simulink library "SingleWorkstationModelLibrary"  (R2014a)
settings: Solver=ode45  StartTime=0.0  StopTime=10.0  RelTol=1e-3
undefined symbols (not defined in the file or in its folder): se_randomizeseeds
(part 2 of 3)

== system SingleWorkstationModelLibrary/GGkWorkstation_MakeAndMoveBatches_Parallel ==
  note: % LICENSE: 3-clause "Revised" or "New" or "Modified" BSD License.
      | % Copyright (c) 2015, Georgia Institute of Technology.
      | % All rights reserved.
      | %
      | % Redistribution and use in source and binary forms, with or without
      | % modification, are permitted provided that the following conditions are met:
      | % * Redistributions of source code must retain the above copyright
      | % notice, this list of conditions and the following disclaimer.
      | % * Redistributions in binary form must reproduce the above copyright
      | % notice, this list of conditions and the following disclaimer in the
      | % documentation and/or other materials provided with the distribution.
      | % * Neither the name of the Georgia Institute of Technology nor the
      | % names of its contributors may be used to endorse or promote products
      | % derived from this software without specific prior written permission.
      | %
      | % THIS SOFTWARE IS PROVIDED BY THE COPYRIGHT HOLDERS AND CONTRIBUTORS "AS IS" AND
      | % ANY EXPRESS OR IMPLIED WARRANTIES, INCLUDING, BUT NOT LIMITED TO, THE IMPLIED
      | % WARRANTIES OF MERCHANTABILITY AND FITNESS FOR A PARTICULAR PURPOSE ARE
      | % DISCLAIMED. IN NO EVENT SHALL THE GEORGIA INSTITUTE OF TECHNOLOGY BE LIABLE FOR
      | % ANY DIRECT, INDIRECT, INCIDENTAL, SPECIAL, EXEMPLARY, OR CONSEQUENTIAL DAMAGES
      | % (INCLUDING, BUT NOT LIMITED TO, PROCUREMENT OF SUBSTITUTE GOODS OR SERVICES;
      | % LOSS OF USE, DATA, OR PROFITS; OR BUSINESS INTERRUPTION) HOWEVER CAUSED AND
      | % ON ANY THEORY OF LIABILITY, WHETHER IN CONTRACT, STRICT LIABILITY, OR TORT
      | % (INCLUDING NEGLIGENCE OR OTHERWISE) ARISING IN ANY WAY OUT OF THE USE OF THIS
      | % SOFTWARE, EVEN IF ADVISED OF THE POSSIBILITY OF SUCH DAMAGE.
  Clock : Clock
  ComputeTH : Subsystem
  ComputeWIP : Subsystem
  GGkWorkstation_MakeAndMoveBatches_Parallel : Subsystem  mask{MakeBatchSize=12, MoveBatchSize=1, NumberOfServers=1}
      mask prompts: MakeBatchSize "Make (a.k.a. Process) Batch Size:"; MoveBatchSize "Move (a.k.a. Transfer) Batch Size"; NumberOfServers "Number of servers:"
      mask Callback MakeBatchSize:
      | %% Capture pre-existing base workspace variables, to cleanup when done
      | preExistingVars = who;
      | 
      | 
      | %% MakeBatchSize is defined as a mask parameter
      | batchSizeStr = get_param(gcbh, 'MakeBatchSize');
      | batchSizeInt = int32(str2double(batchSizeStr));  %Enforce integer
      | if batchSizeInt < 1  %str2double returns NaN for non-numerical input, and int32 returns 0 for NaN
      |     error('Invalid input for MakeBatchSize');
      | end
      | set_param(gcbh, 'MakeBatchSize', num2str(batchSizeInt));  %Correct any non-integer value
      | 
      | 
      | %% Get paths of OutputSwitch, EntityCombiner, EntitySplitter, and PathCombiner
      | singleWksPath = [gcs '/' get(gcbh,'Name')];
      | outputSwitchPath = [singleWksPath '/MakeBatchOutputSwitch'];
      | entityCombinerPath = [singleWksPath '/MakeBatchEntityCombiner'];
      | entitySplitterPath = [singleWksPath '/MakeBatchEntitySplitter'];
      | pathCombinerPath = [singleWksPath '/MakeBatchPathCombiner'];
      | 
      | 
      | %% Unsure if needed:  Disable model library link to enable editing
      | %set_param(singleWksPath, 'LinkStatus', 'inactive');
      | 
      | 
      | %% Delete existing queues and connections
      | phOutputSwitch = get_param(outputSwitchPath, 'PortHandles');
      | phOutputSwitch = phOutputSwitch.RConn;
      | phEntityCombiner = get_param(entityCombinerPath, 'PortHandles');
      | phEntityCombiner = phEntityCombiner.LConn;
      | phEntitySplitter = get_param(entitySplitterPath, 'PortHandles');
      | phEntitySplitter = phEntitySplitter.RConn;
      | 
      | %Delete existing queues
      | oldBatchSize = get_param(outputSwitchPath, 'NumberOutputPorts');
      | queueNamesBeginWith = 'MakeBatchQ';  %Hard-codes a particular naming scheme
      | singleWksBlockList = get(gcbh, 'Blocks');
      | ECQueueMatches = strncmpi(queueNamesBeginWith, singleWksBlockList, length(queueNamesBeginWith));
      | ECQueueNames = singleWksBlockList(ECQueueMatches);
      | if ~isempty(ECQueueNames)
      |     for mm = 1 : length(ECQueueNames)
      |         queuePath = [singleWksPath '/' ECQueueNames{mm}];
      |         queueHandle = get_param(queuePath, 'Handle');
      |         delete(queueHandle);
      |     end
      | end
      | 
      | %Delete the lines
      | for iiiii = 1 : str2double(oldBatchSize)
      |     phOutputSwitchPos = get_param(phOutputSwitch(iiiii), 'Position');
      |     try delete_line(singleWksPath, phOutputSwitchPos); catch, end  %Fail silently
      |     phEntityCombinerPos = get_param(phEntityCombiner(iiiii), 'Position');
      |     try delete_line(singleWksPath, phEntityCombinerPos); catch, end  %Fail silently
      |     phEntitySplitterPos = get_param(phEntitySplitter(iiiii), 'Position');
      |     try delete_line(singleWksPath, phEntitySplitterPos); catch, end  %Fail silently
      | end
      | 
      | 
      | %% Set new number of ports
      | set_param(outputSwitchPath, 'NumberOutputPorts', batchSizeStr);
      | set_param(entityCombinerPath, 'NumberInputPorts', batchSizeStr);
      | set_param(entitySplitterPath, 'NumberOutputPorts', batchSizeStr);
      | set_param(pathCombinerPath, 'NumberInputPorts', batchSizeStr);
      | 
      | 
      | %% Add EntityCombiner input queues, plus connections between OutputSwitch and EntityCombiner
      | phOutputSwitch = get_param(outputSwitchPath, 'PortHandles');
      | phOutputSwitch = phOutputSwitch.RConn;
      | phEntityCombiner = get_param(entityCombinerPath, 'PortHandles');
      | phEntityCombiner = phEntityCombiner.LConn;
      | phEntitySplitter = get_param(entitySplitterPath, 'PortHandles');
      | phEntitySplitter = phEntitySplitter.RConn;
      | phPathCombiner = get_param(pathCombinerPath, 'PortHandles');
      | phPathCombiner = phPathCombiner.LConn;
      | 
      | queueLength = 80;
      | queueHeight = 20;
      | xOffset = 130;
      | prevBlockPos = get_param(outputSwitchPath, 'Position');
      | prevBlockHeight = prevBlockPos(4)-prevBlockPos(2);
      | yIncrement = prevBlockHeight / batchSizeInt;
      | for jjjjj = 1 : batchSizeInt
      |     queuePath = [singleWksPath '/' queueNamesBeginWith num2str(jjjjj)];
      |     queueHandle = add_block('built-in/FIFOQueue', queuePath);
      |     set_param(queueHandle, 'Capacity', 'Inf');  %Shouldn't be needed, but a good default
      | 
      |     left = prevBlockPos(1)+xOffset;
      |     top = double( prevBlockPos(2)+(jjjjj-1)*yIncrement );
      |     right = prevBlockPos(1)+xOffset+queueLength;
      |     bottom = double( prevBlockPos(2)+(jjjjj-1)*yIncrement+queueHeight );
      |     p = [left top right bottom];
      |     set_param(queueHandle, 'Position', p);  %Need a vector of doubles (not int32)
      | 
      |     QueuePortHandles = get_param(queueHandle, 'PortHandles');
      |     %Line from OutputSwitch to Queue
      |     OutputSwitchOutPortPos = get_param(phOutputSwitch(jjjjj), 'Position');
      |     QueueInPortPos = get_param(QueuePortHandles.LConn, 'Position');
      |     add_line(singleWksPath, [OutputSwitchOutPortPos; QueueInPortPos]);
      |     %Line from Queue to EntityCombiner
      |     QueueOutPortPos = get_param(QueuePortHandles.RConn, 'Position');
      |     EntityCombinerInPortPos = get_param(phEntityCombiner(jjjjj), 'Position');
      |     add_line(singleWksPath, [QueueOutPortPos; EntityCombinerInPortPos]);
      | end
      | 
      | 
      | %% Add connections between EntitySplitter and PathCombiner
      | for kkkkk = 1 : batchSizeInt
      |     phEntitySplitterPos = get_param(phEntitySplitter(kkkkk), 'Position');
      |     phPathCombinerPos = get_param(phPathCombiner(kkkkk), 'Position');
      |     add_line(singleWksPath, [phEntitySplitterPos; phPathCombinerPos]);
      | end
      | 
      | 
      | %% Cleanup, because mask callback executes in base workspace
      | clearvars('-except', preExistingVars{:});
      mask Callback MoveBatchSize:
      | %% Capture pre-existing base workspace variables, to cleanup when done
      | preExistingVars = who;
      | 
      | 
      | %% MoveBatchSize is defined as a mask parameter
      | batchSizeStr = get_param(gcbh, 'MoveBatchSize');
      | batchSizeInt = int32(str2double(batchSizeStr));  %Enforce integer
      | if batchSizeInt < 1  %str2double returns NaN for non-numerical input, and int32 returns 0 for NaN
      |     error('Invalid input for MoveBatchSize');
      | end
      | set_param(gcbh, 'MoveBatchSize', num2str(batchSizeInt));  %Correct any non-integer value
      | 
      | 
      | %% Get paths of OutputSwitch, EntityCombiner, EntitySplitter, and PathCombiner
      | singleWksPath = [gcs '/' get(gcbh,'Name')];
      | outputSwitchPath = [singleWksPath '/MoveBatchOutputSwitch'];
      | entityCombinerPath = [singleWksPath '/MoveBatchEntityCombiner'];
      | entitySplitterPath = [singleWksPath '/MoveBatchEntitySplitter'];
      | pathCombinerPath = [singleWksPath '/MoveBatchPathCombiner'];
      | 
      | 
      | %% Unsure if needed:  Disable model library link to enable editing
      | %set_param(singleWksPath, 'LinkStatus', 'inactive');
      | 
      | 
      | %% Delete existing queues and connections
      | phOutputSwitch = get_param(outputSwitchPath, 'PortHandles');
      | phOutputSwitch = phOutputSwitch.RConn;
      | phEntityCombiner = get_param(entityCombinerPath, 'PortHandles');
      | phEntityCombiner = phEntityCombiner.LConn;
      | phEntitySplitter = get_param(entitySplitterPath, 'PortHandles');
      | phEntitySplitter = phEntitySplitter.RConn;
      | 
      | %Delete existing queues
      | oldBatchSize = get_param(outputSwitchPath, 'NumberOutputPorts');
      | queueNamesBeginWith = 'MoveBatchQ';  %Hard-codes a particular naming scheme
      | singleWksBlockList = get(gcbh, 'Blocks');
      | ECQueueMatches = strncmpi(queueNamesBeginWith, singleWksBlockList, length(queueNamesBeginWith));
      | ECQueueNames = singleWksBlockList(ECQueueMatches);
      | if ~isempty(ECQueueNames)
      |     for mm = 1 : length(ECQueueNames)
      |         queuePath = [singleWksPath '/' ECQueueNames{mm}];
      |         queueHandle = get_param(queuePath, 'Handle');
      |         delete(queueHandle);
      |     end
      | end
      | 
      | %Delete the lines
      | for iiiii = 1 : str2double(oldBatchSize)
      |     phOutputSwitchPos = get_param(phOutputSwitch(iiiii), 'Position');
      |     try delete_line(singleWksPath, phOutputSwitchPos); catch, end  %Fail silently
      |     phEntityCombinerPos = get_param(phEntityCombiner(iiiii), 'Position');
      |     try delete_line(singleWksPath, phEntityCombinerPos); catch, end  %Fail silently
      |     phEntitySplitterPos = get_param(phEntitySplitter(iiiii), 'Position');
      |     try delete_line(singleWksPath, phEntitySplitterPos); catch, end  %Fail silently
      | end
      | 
      | 
      | %% Set new number of ports
      | set_param(outputSwitchPath, 'NumberOutputPorts', batchSizeStr);
      | set_param(entityCombinerPath, 'NumberInputPorts', batchSizeStr);
      | set_param(entitySplitterPath, 'NumberOutputPorts', batchSizeStr);
      | set_param(pathCombinerPath, 'NumberInputPorts', batchSizeStr);
      | 
      | 
      | %% Add EntityCombiner input queues, plus connections between OutputSwitch and EntityCombiner
      | phOutputSwitch = get_param(outputSwitchPath, 'PortHandles');
      | phOutputSwitch = phOutputSwitch.RConn;
      | phEntityCombiner = get_param(entityCombinerPath, 'PortHandles');
      | phEntityCombiner = phEntityCombiner.LConn;
      | phEntitySplitter = get_param(entitySplitterPath, 'PortHandles');
      | phEntitySplitter = phEntitySplitter.RConn;
      | phPathCombiner = get_param(pathCombinerPath, 'PortHandles');
      | phPathCombiner = phPathCombiner.LConn;
      | 
      | queueLength = 80;
      | queueHeight = 20;
      | xOffset = 130;
      | prevBlockPos = get_param(outputSwitchPath, 'Position');
      | prevBlockHeight = prevBlockPos(4)-prevBlockPos(2);
      | yIncrement = prevBlockHeight / batchSizeInt;
      | for jjjjj = 1 : batchSizeInt
      |     queuePath = [singleWksPath '/' queueNamesBeginWith num2str(jjjjj)];
      |     queueHandle = add_block('built-in/FIFOQueue', queuePath);
      |     set_param(queueHandle, 'Capacity', 'Inf');
      | 
      | 	left = prevBlockPos(1)+xOffset;
      |     top = double( prevBlockPos(2)+(jjjjj-1)*yIncrement );
      |     right = prevBlockPos(1)+xOffset+queueLength;
      |     bottom = double( prevBlockPos(2)+(jjjjj-1)*yIncrement+queueHeight );
      |     p = [left top right bottom];
      |     set_param(queueHandle, 'Position', p);  %Need a vector of doubles (not int32)
      | 
      |     QueuePortHandles = get_param(queueHandle, 'PortHandles');
      |     %Line from OutputSwitch to Queue
      |     OutputSwitchOutPortPos = get_param(phOutputSwitch(jjjjj), 'Position');
      |     QueueInPortPos = get_param(QueuePortHandles.LConn, 'Position');
      |     add_line(singleWksPath, [OutputSwitchOutPortPos; QueueInPortPos]);
      |     %Line from Queue to EntityCombiner
      |     QueueOutPortPos = get_param(QueuePortHandles.RConn, 'Position');
      |     EntityCombinerInPortPos = get_param(phEntityCombiner(jjjjj), 'Position');
      |     add_line(singleWksPath, [QueueOutPortPos; EntityCombinerInPortPos]);
      | end
      | 
      | 
      | %% Add connections between EntitySplitter and PathCombiner
      | for kkkkk = 1 : batchSizeInt
      |     phEntitySplitterPos = get_param(phEntitySplitter(kkkkk), 'Position');
      |     phPathCombinerPos = get_param(phPathCombiner(kkkkk), 'Position');
      |     add_line(singleWksPath, [phEntitySplitterPos; phPathCombinerPos]);
      | end
      | 
      | 
      | %% Cleanup, because mask callback executes in base workspace
      | clearvars('-except', preExistingVars{:});
      mask TypeOptions NumberOfServers: N-Server/NumberOfServers
      mask DialogControl DescTextVar Prompt: GGk Workstation with Make and Move Batches.  This model implements parallel batch processing, meaning Processing Time is for an entire make (a.k.a. process) batch.  Tokens are output only after a full move (a.k.a. transfer) batch is assembled, and are output individually (as individual entities, not as a batch entity).
  RandomNumbers_ProcessingTimes : EventBasedRandomNumber  meanExp=90  minUnif=40  maxUnif=40  pOneBern=40  pSuccessBino=40  numTrialBino=40  minTri=40  maxTri=40  modeTri=40  thresholdGam=40  scaleGam=40  shapeGam=40  meanNorm=90  stdNorm=eps  pSuccessGeo=40  meanPoiss=40  thresholdLogn=40  scaleLogn=40  shapeLogn=40  thresholdLogl=40  scaleLogl=40  minBeta=40  maxBeta=40  shape1Beta=40  shape2Beta=40  minUnid=40  maxUnid=40  numValueUnid=40  thresholdWbl=40  scaleWbl=40  shapeWbl=40  valueVecCont=40  cdfVecCont=40  valueVecDisc=40  probVecDisc=40  Seed=42055
  Arrivals : PMIOPort  Port=1  Side=Left
  Departures : PMIOPort  Port=2  Side=Right
  WIP_samples : Outport
  WIP_average : Outport  Port=2
  CT_samples : Outport  Port=3
  CT_average : Outport  Port=4
  TH_samples : Outport  Port=5
  TH_average : Outport  Port=6
  Util_average : Outport  Port=7
  wires:
  GGkWorkstation_MakeAndMoveBatches_Parallel/5(Util_average) -> Util_average/1
  GGkWorkstation_MakeAndMoveBatches_Parallel/2(nDepartures) -> ComputeWIP/2(nDepartures), ComputeTH/2(nDepartures)
  GGkWorkstation_MakeAndMoveBatches_Parallel/3(CT_samples) -> CT_samples/1
  GGkWorkstation_MakeAndMoveBatches_Parallel/4(CT_average) -> CT_average/1
  ComputeWIP/1(WIP_samples) -> WIP_samples/1
  ComputeWIP/2(WIP_average) -> WIP_average/1
  GGkWorkstation_MakeAndMoveBatches_Parallel/1(nArrivals) -> ComputeWIP/1(nArrivals)
  Clock/1 -> ComputeWIP/3(CurrentTime), ComputeTH/1(CurrentTime)
  ComputeTH/1(TH_average) -> TH_average/1
  ComputeTH/2(TH_samples) -> TH_samples/1
  RandomNumbers_ProcessingTimes/1 -> GGkWorkstation_MakeAndMoveBatches_Parallel/1(ProcessingTimes)
  connections:
  Departures/RConn1 -- GGkWorkstation_MakeAndMoveBatches_Parallel/RConn1
  GGkWorkstation_MakeAndMoveBatches_Parallel/LConn1 -- Arrivals/RConn1

== system SingleWorkstationModelLibrary/GG1Workstation_FailuresAndSetups/ComputeTH ==
  CurrentTime : Inport
  nDepartures : Inport  Port=2
  Derivative : Derivative
  Divide1 : Product  Inputs=/*
  Event to Timed Signal1 : EventToTimedSignal
  TH_average : Outport
  TH_samples : Outport  Port=2
  wires:
  CurrentTime/1 -> Divide1/1
  Event to Timed Signal1/1 -> Derivative/1, Divide1/2
  Divide1/1 -> TH_average/1
  Derivative/1 -> TH_samples/1
  nDepartures/1 -> Event to Timed Signal1/1

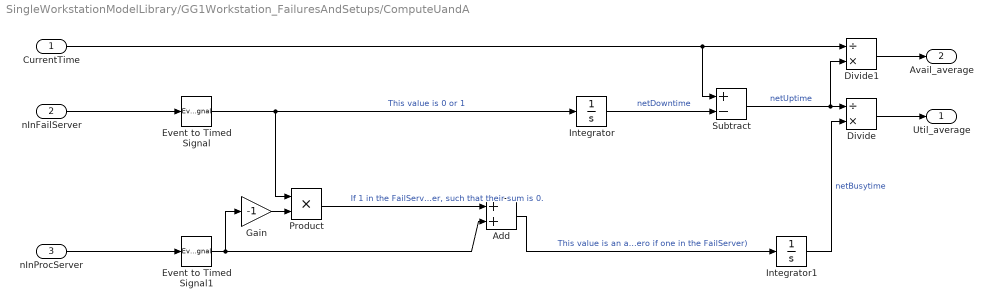
== system SingleWorkstationModelLibrary/GG1Workstation_FailuresAndSetups/ComputeUandA ==
  CurrentTime : Inport
  nInFailServer : Inport  Port=2
  nInProcServer : Inport  Port=3
  Add : Sum
  Divide : Product  Inputs=/*
  Divide1 : Product  Inputs=/*
  Event to Timed Signal : EventToTimedSignal
  Event to Timed Signal1 : EventToTimedSignal
  Gain : Gain  Gain=-1
  Integrator : Integrator
  Integrator1 : Integrator
  Product : Product
  Subtract : Sum  Inputs=+-
  Util_average : Outport
  Avail_average : Outport  Port=2
  wires:
  Event to Timed Signal/1 -> Integrator/1, Product/1  "This value is 0 or 1"
  nInFailServer/1 -> Event to Timed Signal/1
  nInProcServer/1 -> Event to Timed Signal1/1
  Integrator/1 -> Subtract/2  "netDowntime"
  CurrentTime/1 -> Subtract/1, Divide1/1
  Divide/1 -> Util_average/1
  Subtract/1 -> Divide/1, Divide1/2  "netUptime"
  Integrator1/1 -> Divide/2  "netBusytime"
  Gain/1 -> Product/2
  Product/1 -> Add/1  "If 1 in the FailServer, then this value should be negative the number in the ProcServer, such that their sum is 0."
  Add/1 -> Integrator1/1  "This value is an adjusted number in the ProcServer (zero if one in the FailServer)"
  Event to Timed Signal1/1 -> Add/2, Gain/1
  Divide1/1 -> Avail_average/1

== system SingleWorkstationModelLibrary/GG1Workstation_FailuresAndSetups/ComputeWIP ==
  nArrivals : Inport
  nDepartures : Inport  Port=2
  CurrentTime : Inport  Port=3
  Divide : Product  Inputs=*/
  Event to Timed Signal : EventToTimedSignal
  Integrator : Integrator
  Subtract : Sum  Inputs=+-
  WIP_samples : Outport
  WIP_average : Outport  Port=2
  wires:
  Subtract/1 -> WIP_samples/1, Event to Timed Signal/1
  Event to Timed Signal/1 -> Integrator/1
  Divide/1 -> WIP_average/1
  Integrator/1 -> Divide/1
  nArrivals/1 -> Subtract/1
  nDepartures/1 -> Subtract/2
  CurrentTime/1 -> Divide/2

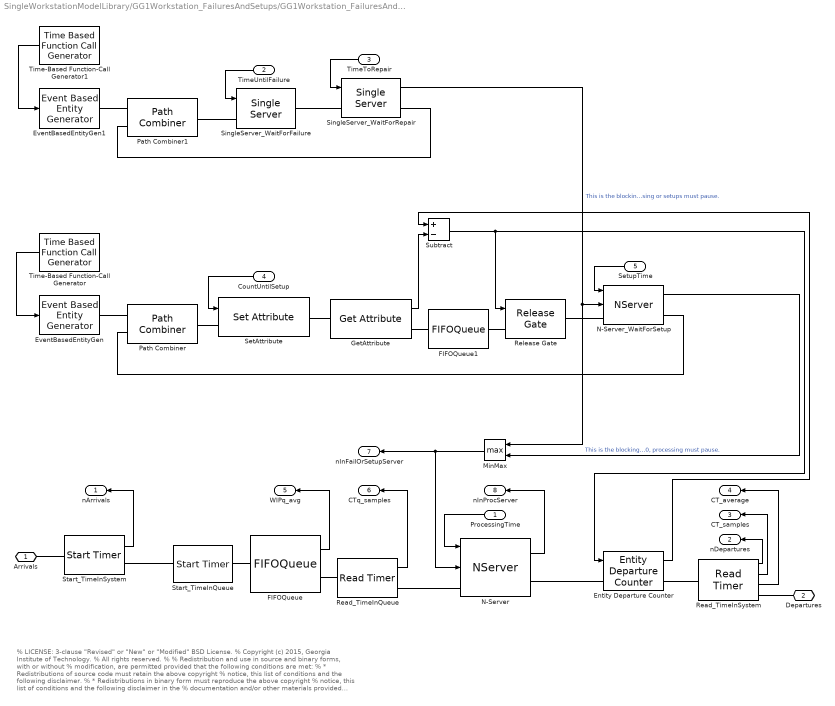
== system SingleWorkstationModelLibrary/GG1Workstation_FailuresAndSetups/GG1Workstation_FailuresAndSetups ==
  note: % LICENSE: 3-clause "Revised" or "New" or "Modified" BSD License.
      | % Copyright (c) 2015, Georgia Institute of Technology.
      | % All rights reserved.
      | %
      | % Redistribution and use in source and binary forms, with or without
      | % modification, are permitted provided that the following conditions are met:
      | % * Redistributions of source code must retain the above copyright
      | % notice, this list of conditions and the following disclaimer.
      | % * Redistributions in binary form must reproduce the above copyright
      | % notice, this list of conditions and the following disclaimer in the
      | % documentation and/or other materials provided with the distribution.
      | % * Neither the name of the Georgia Institute of Technology nor the
      | % names of its contributors may be used to endorse or promote products
      | % derived from this software without specific prior written permission.
      | %
      | % THIS SOFTWARE IS PROVIDED BY THE COPYRIGHT HOLDERS AND CONTRIBUTORS "AS IS" AND
      | % ANY EXPRESS OR IMPLIED WARRANTIES, INCLUDING, BUT NOT LIMITED TO, THE IMPLIED
      | % WARRANTIES OF MERCHANTABILITY AND FITNESS FOR A PARTICULAR PURPOSE ARE
      | % DISCLAIMED. IN NO EVENT SHALL THE GEORGIA INSTITUTE OF TECHNOLOGY BE LIABLE FOR
      | % ANY DIRECT, INDIRECT, INCIDENTAL, SPECIAL, EXEMPLARY, OR CONSEQUENTIAL DAMAGES
      | % (INCLUDING, BUT NOT LIMITED TO, PROCUREMENT OF SUBSTITUTE GOODS OR SERVICES;
      | % LOSS OF USE, DATA, OR PROFITS; OR BUSINESS INTERRUPTION) HOWEVER CAUSED AND
      | % ON ANY THEORY OF LIABILITY, WHETHER IN CONTRACT, STRICT LIABILITY, OR TORT
      | % (INCLUDING NEGLIGENCE OR OTHERWISE) ARISING IN ANY WAY OUT OF THE USE OF THIS
      | % SOFTWARE, EVEN IF ADVISED OF THE POSSIBILITY OF SUCH DAMAGE.
  ProcessingTime : Inport
  TimeUntilFailure : Inport  Port=2
  TimeToRepair : Inport  Port=3
  CountUntilSetup : Inport  Port=4
  SetupTime : Inport  Port=5
  Entity Departure Counter : EntityDepartureCounter  NumberDepartedToSignal=on  NumberDepartedToAttribute=off  CounterResetTypeOption=Trigger from port tr
  EventBasedEntityGen : EventBasedEntityGenerator  GenerateEntitiesUpon=Function call from port fcn
  EventBasedEntityGen1 : EventBasedEntityGenerator  GenerateEntitiesUpon=Function call from port fcn
  FIFOQueue : FIFOQueue  Capacity=Capacity  StatAverageQueueLength=on
      settings: OutputPortMap=o3
  FIFOQueue1 : FIFOQueue  Capacity=Inf
  GetAttribute : GetAttribute  AttributeName=CountUntilSetup  EvaluatedDefaultAttributeValue={ []}
      settings: OutputPortMap=o1
  MinMax : MinMax  Function=max  Inputs=2
  N-Server : NServer  NumberOfServers=1  ServiceTimeFrom=Signal port t  AllowServiceControl=on  BlockWhileSignalOn=on  StatNumberInBlock=on
      settings: InputPortMap=u0,u1  OutputPortMap=o1
  N-Server_WaitForSetup : NServer  NumberOfServers=1  ServiceTimeFrom=Signal port t  AllowServiceControl=on  BlockWhileSignalOn=on  StatNumberInBlock=on
      settings: InputPortMap=u0,u1  OutputPortMap=o1
  Path Combiner : PathCombiner  NumberInputPorts=2
  Path Combiner1 : PathCombiner  NumberInputPorts=2
  Read_TimeInQueue : ReadTimer  TimerTag=TimeInQueue  StatTimeElapsed=on
      settings: OutputPortMap=o2
  Read_TimeInSystem : ReadTimer  TimerTag=TimeInSystem  StatNumberDeparted=on  StatTimeElapsed=on  StatAverageTimeElapsed=on
      settings: OutputPortMap=o0,o2,o3
  Release Gate : ReleaseGate  OpenGateUpon=Trigger from port tr
  SetAttribute : SetAttribute  AttributeName=CountUntilSetup  AttributeFrom=Signal port  EvaluatedAttributeValue={ []}
  SingleServer_WaitForFailure : SingleServer  ServiceTimeFrom=Signal port t  AttributeName=TimeUntilFailure
  SingleServer_WaitForRepair : SingleServer  ServiceTimeFrom=Signal port t  AttributeName=TimeToRepair  StatNumberInBlock=on
      settings: OutputPortMap=o1
  Start_TimeInQueue : StartTimer  TimerTag=TimeInQueue  TimerStartedOption=Restart
  Start_TimeInSystem : StartTimer  TimerTag=TimeInSystem  TimerStartedOption=Restart  StatNumberDeparted=on
  Subtract : Sum  Inputs=+-
  Time-Based Function-Call Generator : TimeBasedFunctionCallGenerator  EventGenerationMode=Only at simulation start
  Time-Based Function-Call Generator1 : TimeBasedFunctionCallGenerator  EventGenerationMode=Only at simulation start
  Arrivals : PMIOPort  Port=1  Side=Left
  Departures : PMIOPort  Port=2  Side=Right
  nArrivals : Outport
  nDepartures : Outport  Port=2
  CT_samples : Outport  Port=3
  CT_average : Outport  Port=4
  WIPq_avg : Outport  Port=5
  CTq_samples : Outport  Port=6
  nInFailOrSetupServer : Outport  Port=7
  nInProcServer : Outport  Port=8
  wires:
  Read_TimeInSystem/2 -> CT_samples/1
  Read_TimeInQueue/1 -> CTq_samples/1
  FIFOQueue/1 -> WIPq_avg/1
  Start_TimeInSystem/1 -> nArrivals/1
  Read_TimeInSystem/1 -> nDepartures/1
  ProcessingTime/1 -> N-Server/1
  Read_TimeInSystem/3 -> CT_average/1
  Time-Based Function-Call Generator/1 -> EventBasedEntityGen/1
  CountUntilSetup/1 -> SetAttribute/1
  Subtract/1 -> Release Gate/1, Entity Departure Counter/1
  GetAttribute/1 -> Subtract/2
  Entity Departure Counter/1 -> Subtract/1
  N-Server/1 -> nInProcServer/1
  SetupTime/1 -> N-Server_WaitForSetup/1
  Time-Based Function-Call Generator1/1 -> EventBasedEntityGen1/1
  TimeToRepair/1 -> SingleServer_WaitForRepair/1
  TimeUntilFailure/1 -> SingleServer_WaitForFailure/1
  SingleServer_WaitForRepair/1 -> MinMax/1, N-Server_WaitForSetup/2  "This is the blocking signal from failures. When >0, processing or setups must pause."
  N-Server_WaitForSetup/1 -> MinMax/2  "This is the blocking signal from setups.  When >0, processing must pause."
  MinMax/1 -> nInFailOrSetupServer/1, N-Server/2
  connections:
  Arrivals/RConn1 -- Start_TimeInSystem/LConn1
  FIFOQueue/RConn1 -- Read_TimeInQueue/LConn1
  Start_TimeInSystem/RConn1 -- Start_TimeInQueue/LConn1
  Read_TimeInSystem/RConn1 -- Departures/RConn1
  Read_TimeInQueue/RConn1 -- N-Server/LConn1
  Start_TimeInQueue/RConn1 -- FIFOQueue/LConn1
  Path Combiner/RConn1 -- SetAttribute/LConn1
  EventBasedEntityGen/RConn1 -- Path Combiner/LConn1
  Path Combiner/LConn2 -- N-Server_WaitForSetup/RConn1
  N-Server/RConn1 -- Entity Departure Counter/LConn1
  Entity Departure Counter/RConn1 -- Read_TimeInSystem/LConn1
  FIFOQueue1/LConn1 -- GetAttribute/RConn1
  N-Server_WaitForSetup/LConn1 -- Release Gate/RConn1
  FIFOQueue1/RConn1 -- Release Gate/LConn1
  SetAttribute/RConn1 -- GetAttribute/LConn1
  Path Combiner1/LConn2 -- SingleServer_WaitForRepair/RConn1
  SingleServer_WaitForRepair/LConn1 -- SingleServer_WaitForFailure/RConn1
  EventBasedEntityGen1/RConn1 -- Path Combiner1/LConn1
  Path Combiner1/RConn1 -- SingleServer_WaitForFailure/LConn1

== system SingleWorkstationModelLibrary/GG1Workstation_MakeAndMoveBatches_SerialWithSetups/ComputeTH ==
  CurrentTime : Inport
  nDepartures : Inport  Port=2
  Derivative : Derivative
  Divide1 : Product  Inputs=/*
  Event to Timed Signal1 : EventToTimedSignal
  TH_average : Outport
  TH_samples : Outport  Port=2
  wires:
  CurrentTime/1 -> Divide1/1
  Event to Timed Signal1/1 -> Derivative/1, Divide1/2
  Divide1/1 -> TH_average/1
  Derivative/1 -> TH_samples/1
  nDepartures/1 -> Event to Timed Signal1/1

== system SingleWorkstationModelLibrary/GG1Workstation_MakeAndMoveBatches_SerialWithSetups/ComputeWIP ==
  nArrivals : Inport
  nDepartures : Inport  Port=2
  CurrentTime : Inport  Port=3
  Divide : Product  Inputs=*/
  Event to Timed Signal : EventToTimedSignal
  Integrator : Integrator
  Subtract : Sum  Inputs=+-
  WIP_samples : Outport
  WIP_average : Outport  Port=2
  wires:
  Subtract/1 -> WIP_samples/1, Event to Timed Signal/1
  Event to Timed Signal/1 -> Integrator/1
  Divide/1 -> WIP_average/1
  Integrator/1 -> Divide/1
  nArrivals/1 -> Subtract/1
  nDepartures/1 -> Subtract/2
  CurrentTime/1 -> Divide/2

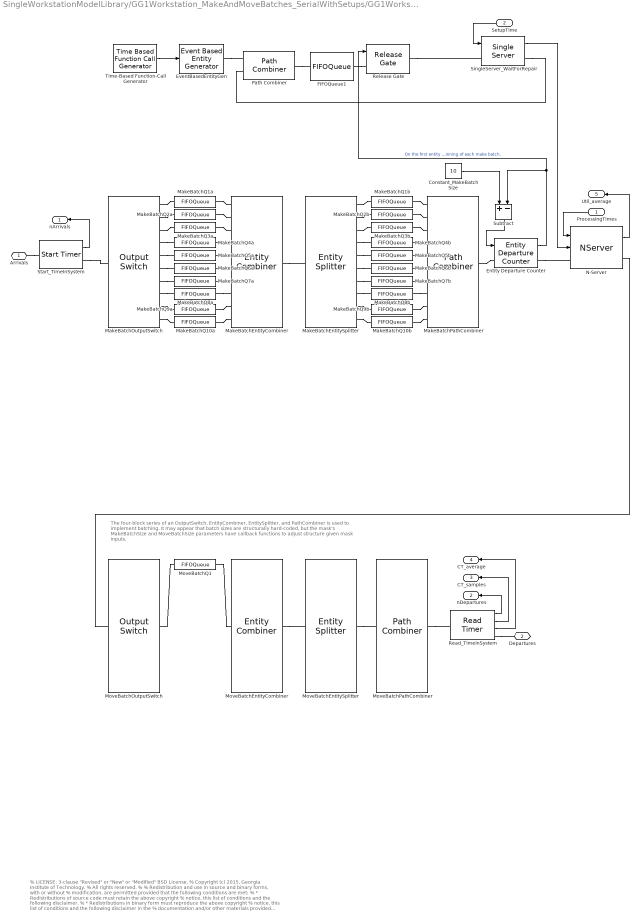
== system SingleWorkstationModelLibrary/GG1Workstation_MakeAndMoveBatches_SerialWithSetups/GG1Workstation_MakeAndMoveBatches_SerialWithSetups ==
  note: The four-block series of an OutputSwitch, EntityCombiner, EntitySplitter, and PathCombiner is used
      | to implement batching. It may appear that batch sizes are structurally hard-coded, but the mask's
      | MakeBatchSize and MoveBatchSize parameters have callback functions to adjust structure given
      | mask inputs.
  note: % LICENSE: 3-clause "Revised" or "New" or "Modified" BSD License.
      | % Copyright (c) 2015, Georgia Institute of Technology.
      | % All rights reserved.
      | %
      | % Redistribution and use in source and binary forms, with or without
      | % modification, are permitted provided that the following conditions are met:
      | % * Redistributions of source code must retain the above copyright
      | % notice, this list of conditions and the following disclaimer.
      | % * Redistributions in binary form must reproduce the above copyright
      | % notice, this list of conditions and the following disclaimer in the
      | % documentation and/or other materials provided with the distribution.
      | % * Neither the name of the Georgia Institute of Technology nor the
      | % names of its contributors may be used to endorse or promote products
      | % derived from this software without specific prior written permission.
      | %
      | % THIS SOFTWARE IS PROVIDED BY THE COPYRIGHT HOLDERS AND CONTRIBUTORS "AS IS" AND
      | % ANY EXPRESS OR IMPLIED WARRANTIES, INCLUDING, BUT NOT LIMITED TO, THE IMPLIED
      | % WARRANTIES OF MERCHANTABILITY AND FITNESS FOR A PARTICULAR PURPOSE ARE
      | % DISCLAIMED. IN NO EVENT SHALL THE GEORGIA INSTITUTE OF TECHNOLOGY BE LIABLE FOR
      | % ANY DIRECT, INDIRECT, INCIDENTAL, SPECIAL, EXEMPLARY, OR CONSEQUENTIAL DAMAGES
      | % (INCLUDING, BUT NOT LIMITED TO, PROCUREMENT OF SUBSTITUTE GOODS OR SERVICES;
      | % LOSS OF USE, DATA, OR PROFITS; OR BUSINESS INTERRUPTION) HOWEVER CAUSED AND
      | % ON ANY THEORY OF LIABILITY, WHETHER IN CONTRACT, STRICT LIABILITY, OR TORT
      | % (INCLUDING NEGLIGENCE OR OTHERWISE) ARISING IN ANY WAY OUT OF THE USE OF THIS
      | % SOFTWARE, EVEN IF ADVISED OF THE POSSIBILITY OF SUCH DAMAGE.
  ProcessingTimes : Inport
  SetupTime : Inport  Port=2
  Constant_MakeBatchSize : Constant  Value=10
  Entity Departure Counter : EntityDepartureCounter  NumberDepartedToSignal=on  NumberDepartedToAttribute=off  CounterResetTypeOption=Trigger from port tr  CounterResetEdgeOption=Falling
  EventBasedEntityGen : EventBasedEntityGenerator  GenerateEntitiesUpon=Function call from port fcn
  FIFOQueue1 : FIFOQueue  Capacity=Inf
  MakeBatchEntityCombiner : EntityCombiner  NumberInputPorts=10  AttributeAccessibility=off  TimerAccessibility=off
  MakeBatchEntitySplitter : EntitySplitter  NumberOutputPorts=10
  MakeBatchOutputSwitch : OutputSwitch  NumberOutputPorts=10  SwitchingCriterion=Round robin
  MakeBatchPathCombiner : PathCombiner  NumberInputPorts=10
  MakeBatchQ10a : FIFOQueue  Capacity=Inf
  MakeBatchQ10b : FIFOQueue  Capacity=1
  MakeBatchQ1a : FIFOQueue  Capacity=Inf
  MakeBatchQ1b : FIFOQueue  Capacity=1
  MakeBatchQ2a : FIFOQueue  Capacity=Inf
  MakeBatchQ2b : FIFOQueue  Capacity=1
  MakeBatchQ3a : FIFOQueue  Capacity=Inf
  MakeBatchQ3b : FIFOQueue  Capacity=1
  MakeBatchQ4a : FIFOQueue  Capacity=Inf
  MakeBatchQ4b : FIFOQueue  Capacity=1
  MakeBatchQ5a : FIFOQueue  Capacity=Inf
  MakeBatchQ5b : FIFOQueue  Capacity=1
  MakeBatchQ6a : FIFOQueue  Capacity=Inf
  MakeBatchQ6b : FIFOQueue  Capacity=1
  MakeBatchQ7a : FIFOQueue  Capacity=Inf
  MakeBatchQ7b : FIFOQueue  Capacity=1
  MakeBatchQ8a : FIFOQueue  Capacity=Inf
  MakeBatchQ8b : FIFOQueue  Capacity=1
  MakeBatchQ9a : FIFOQueue  Capacity=Inf
  MakeBatchQ9b : FIFOQueue  Capacity=1
  MoveBatchEntityCombiner : EntityCombiner  NumberInputPorts=1  AttributeAccessibility=off  TimerAccessibility=off
  MoveBatchEntitySplitter : EntitySplitter  NumberOutputPorts=1
  MoveBatchOutputSwitch : OutputSwitch  NumberOutputPorts=1  SwitchingCriterion=Round robin
  MoveBatchPathCombiner : PathCombiner  NumberInputPorts=1
  MoveBatchQ1 : FIFOQueue  Capacity=1
  N-Server : NServer  NumberOfServers=1  ServiceTimeFrom=Signal port t  AllowServiceControl=on  StatUtilization=on
      settings: InputPortMap=u0,u1  OutputPortMap=o5
  Path Combiner : PathCombiner  NumberInputPorts=2
  Read_TimeInSystem : ReadTimer  TimerTag=TimeInSystem  StatNumberDeparted=on  StatTimeElapsed=on  StatAverageTimeElapsed=on
      settings: OutputPortMap=o0,o2,o3
  Release Gate : ReleaseGate  OpenGateUpon=Trigger from port tr
  SingleServer_WaitForRepair : SingleServer  ServiceTimeFrom=Signal port t  AttributeName=SetupTime  StatNumberInBlock=on
      settings: OutputPortMap=o1
  Start_TimeInSystem : StartTimer  TimerTag=TimeInSystem  TimerStartedOption=Restart  StatNumberDeparted=on
  Subtract : Sum  Inputs=+-
  Time-Based Function-Call Generator : TimeBasedFunctionCallGenerator  EventGenerationMode=Only at simulation start
  Arrivals : PMIOPort  Port=1  Side=Left
  Departures : PMIOPort  Port=2  Side=Right
  nArrivals : Outport
  nDepartures : Outport  Port=2
  CT_samples : Outport  Port=3
  CT_average : Outport  Port=4
  Util_average : Outport  Port=5
  wires:
  Start_TimeInSystem/1 -> nArrivals/1
  Read_TimeInSystem/1 -> nDepartures/1
  Read_TimeInSystem/2 -> CT_samples/1
  ProcessingTimes/1 -> N-Server/1
  Read_TimeInSystem/3 -> CT_average/1
  Time-Based Function-Call Generator/1 -> EventBasedEntityGen/1
  SingleServer_WaitForRepair/1 -> N-Server/2
  SetupTime/1 -> SingleServer_WaitForRepair/1
  Entity Departure Counter/1 -> Subtract/2, Release Gate/1  "On the first entity of a make batch, this signal rises from 0 to 1 and triggers the release of a setup entity. The effect is setups which are not count-based, but rather upon the beginning of each make batch."
  Constant_MakeBatchSize/1 -> Subtract/1
  Subtract/1 -> Entity Departure Counter/1
  N-Server/1 -> Util_average/1
  connections:
  Read_TimeInSystem/RConn1 -- Departures/RConn1
  Arrivals/RConn1 -- Start_TimeInSystem/LConn1
  MoveBatchEntityCombiner/RConn1 -- MoveBatchEntitySplitter/LConn1
  Start_TimeInSystem/RConn1 -- MakeBatchOutputSwitch/LConn1
  MoveBatchPathCombiner/RConn1 -- Read_TimeInSystem/LConn1
  EventBasedEntityGen/RConn1 -- Path Combiner/LConn1
  SingleServer_WaitForRepair/RConn1 -- Path Combiner/LConn2
  Release Gate/RConn1 -- SingleServer_WaitForRepair/LConn1
  FIFOQueue1/RConn1 -- Release Gate/LConn1
  MakeBatchEntityCombiner/RConn1 -- MakeBatchEntitySplitter/LConn1
  Path Combiner/RConn1 -- FIFOQueue1/LConn1
  MakeBatchPathCombiner/RConn1 -- Entity Departure Counter/LConn1
  Entity Departure Counter/RConn1 -- N-Server/LConn1
  N-Server/RConn1 -- MoveBatchOutputSwitch/LConn1
  MakeBatchOutputSwitch/RConn1 -- MakeBatchQ1a/LConn1
  MakeBatchQ1a/RConn1 -- MakeBatchEntityCombiner/LConn1
  MakeBatchEntitySplitter/RConn1 -- MakeBatchQ1b/LConn1
  MakeBatchQ1b/RConn1 -- MakeBatchPathCombiner/LConn1
  MakeBatchOutputSwitch/RConn2 -- MakeBatchQ2a/LConn1
  MakeBatchQ2a/RConn1 -- MakeBatchEntityCombiner/LConn2
  MakeBatchEntitySplitter/RConn2 -- MakeBatchQ2b/LConn1
  MakeBatchQ2b/RConn1 -- MakeBatchPathCombiner/LConn2
  MakeBatchOutputSwitch/RConn3 -- MakeBatchQ3a/LConn1
  MakeBatchQ3a/RConn1 -- MakeBatchEntityCombiner/LConn3
  MakeBatchEntitySplitter/RConn3 -- MakeBatchQ3b/LConn1
  MakeBatchQ3b/RConn1 -- MakeBatchPathCombiner/LConn3
  MakeBatchOutputSwitch/RConn4 -- MakeBatchQ4a/LConn1
  MakeBatchQ4a/RConn1 -- MakeBatchEntityCombiner/LConn4
  MakeBatchEntitySplitter/RConn4 -- MakeBatchQ4b/LConn1
  MakeBatchQ4b/RConn1 -- MakeBatchPathCombiner/LConn4
  MakeBatchOutputSwitch/RConn5 -- MakeBatchQ5a/LConn1
  MakeBatchQ5a/RConn1 -- MakeBatchEntityCombiner/LConn5
  MakeBatchEntitySplitter/RConn5 -- MakeBatchQ5b/LConn1
  MakeBatchQ5b/RConn1 -- MakeBatchPathCombiner/LConn5
  MakeBatchOutputSwitch/RConn6 -- MakeBatchQ6a/LConn1
  MakeBatchQ6a/RConn1 -- MakeBatchEntityCombiner/LConn6
  MakeBatchEntitySplitter/RConn6 -- MakeBatchQ6b/LConn1
  MakeBatchQ6b/RConn1 -- MakeBatchPathCombiner/LConn6
  MakeBatchOutputSwitch/RConn7 -- MakeBatchQ7a/LConn1
  MakeBatchQ7a/RConn1 -- MakeBatchEntityCombiner/LConn7
  MakeBatchEntitySplitter/RConn7 -- MakeBatchQ7b/LConn1
  MakeBatchQ7b/RConn1 -- MakeBatchPathCombiner/LConn7
  MakeBatchOutputSwitch/RConn8 -- MakeBatchQ8a/LConn1
  MakeBatchQ8a/RConn1 -- MakeBatchEntityCombiner/LConn8
  MakeBatchEntitySplitter/RConn8 -- MakeBatchQ8b/LConn1
  MakeBatchQ8b/RConn1 -- MakeBatchPathCombiner/LConn8
  MakeBatchOutputSwitch/RConn9 -- MakeBatchQ9a/LConn1
  MakeBatchQ9a/RConn1 -- MakeBatchEntityCombiner/LConn9
  MakeBatchEntitySplitter/RConn9 -- MakeBatchQ9b/LConn1
  MakeBatchQ9b/RConn1 -- MakeBatchPathCombiner/LConn9
  MakeBatchOutputSwitch/RConn10 -- MakeBatchQ10a/LConn1
  MakeBatchQ10a/RConn1 -- MakeBatchEntityCombiner/LConn10
  MakeBatchEntitySplitter/RConn10 -- MakeBatchQ10b/LConn1
  MakeBatchQ10b/RConn1 -- MakeBatchPathCombiner/LConn10
  MoveBatchOutputSwitch/RConn1 -- MoveBatchQ1/LConn1
  MoveBatchQ1/RConn1 -- MoveBatchEntityCombiner/LConn1
  MoveBatchEntitySplitter/RConn1 -- MoveBatchPathCombiner/LConn1

== system SingleWorkstationModelLibrary/GG1Workstation_RandomCalendarTimeUntilPreempFailure/ComputeTH ==
  CurrentTime : Inport
  nDepartures : Inport  Port=2
  Derivative : Derivative
  Divide : Product  Inputs=/*
  Event to Timed Signal : EventToTimedSignal
  TH_average : Outport
  TH_samples : Outport  Port=2
  wires:
  CurrentTime/1 -> Divide/1
  Event to Timed Signal/1 -> Derivative/1, Divide/2
  Divide/1 -> TH_average/1
  Derivative/1 -> TH_samples/1
  nDepartures/1 -> Event to Timed Signal/1

== system SingleWorkstationModelLibrary/GG1Workstation_RandomCalendarTimeUntilPreempFailure/ComputeUandA ==
  CurrentTime : Inport
  nInFailServer : Inport  Port=2
  nInProcServer : Inport  Port=3
  Add : Sum
  Divide : Product  Inputs=/*
  Divide1 : Product  Inputs=/*
  Event to Timed Signal : EventToTimedSignal
  Event to Timed Signal1 : EventToTimedSignal
  Gain : Gain  Gain=-1
  Integrator : Integrator
  Integrator1 : Integrator
  Product : Product
  Subtract : Sum  Inputs=+-
  Util_average : Outport
  Avail_average : Outport  Port=2
  wires:
  Event to Timed Signal/1 -> Integrator/1, Product/1  "This value is 0 or 1"
  nInFailServer/1 -> Event to Timed Signal/1
  nInProcServer/1 -> Event to Timed Signal1/1
  Integrator/1 -> Subtract/2  "netDowntime"
  CurrentTime/1 -> Subtract/1, Divide1/1
  Divide/1 -> Util_average/1
  Subtract/1 -> Divide/1, Divide1/2  "netUptime"
  Integrator1/1 -> Divide/2  "netBusytime"
  Gain/1 -> Product/2
  Product/1 -> Add/1  "If 1 in the FailServer, then this value should be negative the number in the ProcServer, such that their sum is 0."
  Add/1 -> Integrator1/1  "This value is an adjusted number in the ProcServer (zero if one in the FailServer)"
  Event to Timed Signal1/1 -> Add/2, Gain/1
  Divide1/1 -> Avail_average/1

== system SingleWorkstationModelLibrary/GG1Workstation_RandomCalendarTimeUntilPreempFailure/ComputeWIP ==
  nArrivals : Inport
  nDepartures : Inport  Port=2
  CurrentTime : Inport  Port=3
  Divide : Product  Inputs=*/
  Event to Timed Signal : EventToTimedSignal
  Integrator : Integrator
  Subtract : Sum  Inputs=+-
  WIP_samples : Outport
  WIP_average : Outport  Port=2
  wires:
  Subtract/1 -> WIP_samples/1, Event to Timed Signal/1
  Event to Timed Signal/1 -> Integrator/1
  Divide/1 -> WIP_average/1
  Integrator/1 -> Divide/1
  nArrivals/1 -> Subtract/1
  nDepartures/1 -> Subtract/2
  CurrentTime/1 -> Divide/2

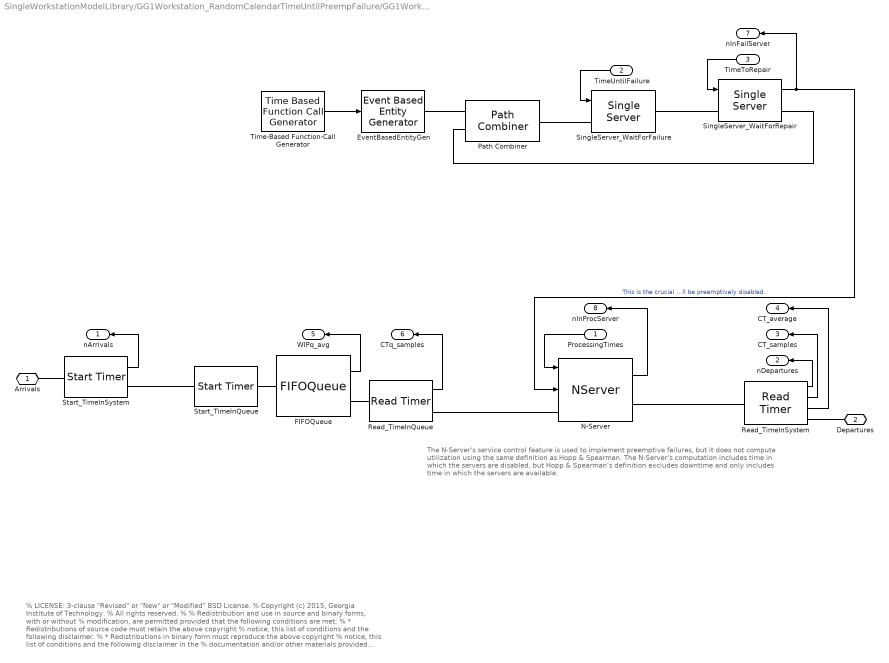
== system SingleWorkstationModelLibrary/GG1Workstation_RandomCalendarTimeUntilPreempFailure/GG1Workstation_RandomCalendarTimeUntilPreempFailure ==
  note: The N-Server's service control feature is used to implement preemptive failures,
      | but it does not compute utilization using the same definition as Hopp & Spearman.
      | The N-Server's computation includes time in which the servers are disabled, but
      | Hopp & Spearman's definition excludes downtime and only includes time in which
      | the servers are available.
  note: % LICENSE: 3-clause "Revised" or "New" or "Modified" BSD License.
      | % Copyright (c) 2015, Georgia Institute of Technology.
      | % All rights reserved.
      | %
      | % Redistribution and use in source and binary forms, with or without
      | % modification, are permitted provided that the following conditions are met:
      | % * Redistributions of source code must retain the above copyright
      | % notice, this list of conditions and the following disclaimer.
      | % * Redistributions in binary form must reproduce the above copyright
      | % notice, this list of conditions and the following disclaimer in the
      | % documentation and/or other materials provided with the distribution.
      | % * Neither the name of the Georgia Institute of Technology nor the
      | % names of its contributors may be used to endorse or promote products
      | % derived from this software without specific prior written permission.
      | %
      | % THIS SOFTWARE IS PROVIDED BY THE COPYRIGHT HOLDERS AND CONTRIBUTORS "AS IS" AND
      | % ANY EXPRESS OR IMPLIED WARRANTIES, INCLUDING, BUT NOT LIMITED TO, THE IMPLIED
      | % WARRANTIES OF MERCHANTABILITY AND FITNESS FOR A PARTICULAR PURPOSE ARE
      | % DISCLAIMED. IN NO EVENT SHALL THE GEORGIA INSTITUTE OF TECHNOLOGY BE LIABLE FOR
      | % ANY DIRECT, INDIRECT, INCIDENTAL, SPECIAL, EXEMPLARY, OR CONSEQUENTIAL DAMAGES
      | % (INCLUDING, BUT NOT LIMITED TO, PROCUREMENT OF SUBSTITUTE GOODS OR SERVICES;
      | % LOSS OF USE, DATA, OR PROFITS; OR BUSINESS INTERRUPTION) HOWEVER CAUSED AND
      | % ON ANY THEORY OF LIABILITY, WHETHER IN CONTRACT, STRICT LIABILITY, OR TORT
      | % (INCLUDING NEGLIGENCE OR OTHERWISE) ARISING IN ANY WAY OUT OF THE USE OF THIS
      | % SOFTWARE, EVEN IF ADVISED OF THE POSSIBILITY OF SUCH DAMAGE.
  ProcessingTimes : Inport
  TimeUntilFailure : Inport  Port=2
  TimeToRepair : Inport  Port=3
  EventBasedEntityGen : EventBasedEntityGenerator  GenerateEntitiesUpon=Function call from port fcn
  FIFOQueue : FIFOQueue  Capacity=Capacity  StatAverageQueueLength=on
      settings: OutputPortMap=o3
  N-Server : NServer  NumberOfServers=1  ServiceTimeFrom=Signal port t  ServiceTime=0  AttributeName=ProcTime  AllowServiceControl=on  BlockWhileSignalOn=on  StatNumberInBlock=on
      settings: InputPortMap=u0,u1  OutputPortMap=o1
  Path Combiner : PathCombiner  NumberInputPorts=2
  Read_TimeInQueue : ReadTimer  TimerTag=TimeInQueue  StatTimeElapsed=on
      settings: OutputPortMap=o2
  Read_TimeInSystem : ReadTimer  TimerTag=TimeInSystem  StatNumberDeparted=on  StatTimeElapsed=on  StatAverageTimeElapsed=on
      settings: OutputPortMap=o0,o2,o3
  SingleServer_WaitForFailure : SingleServer  ServiceTimeFrom=Signal port t  AttributeName=TimeUntilFailure
  SingleServer_WaitForRepair : SingleServer  ServiceTimeFrom=Signal port t  AttributeName=TimeToRepair  StatNumberInBlock=on
      settings: OutputPortMap=o1
  Start_TimeInQueue : StartTimer  TimerTag=TimeInQueue  TimerStartedOption=Restart
  Start_TimeInSystem : StartTimer  TimerTag=TimeInSystem  TimerStartedOption=Restart  StatNumberDeparted=on
  Time-Based Function-Call Generator : TimeBasedFunctionCallGenerator  EventGenerationMode=Only at simulation start
  Arrivals : PMIOPort  Port=1  Side=Left
  Departures : PMIOPort  Port=2  Side=Right
  nArrivals : Outport
  nDepartures : Outport  Port=2
  CT_samples : Outport  Port=3
  CT_average : Outport  Port=4
  WIPq_avg : Outport  Port=5
  CTq_samples : Outport  Port=6
  nInFailServer : Outport  Port=7
  nInProcServer : Outport  Port=8
  wires:
  Read_TimeInSystem/2 -> CT_samples/1
  Read_TimeInQueue/1 -> CTq_samples/1
  FIFOQueue/1 -> WIPq_avg/1
  Start_TimeInSystem/1 -> nArrivals/1
  Read_TimeInSystem/1 -> nDepartures/1
  Read_TimeInSystem/3 -> CT_average/1
  Time-Based Function-Call Generator/1 -> EventBasedEntityGen/1
  SingleServer_WaitForRepair/1 -> N-Server/2, nInFailServer/1  "This is the crucial blocking signal. When > 0, the N-Server will be preemptively disabled."
  ProcessingTimes/1 -> N-Server/1
  N-Server/1 -> nInProcServer/1
  TimeToRepair/1 -> SingleServer_WaitForRepair/1
  TimeUntilFailure/1 -> SingleServer_WaitForFailure/1
  connections:
  FIFOQueue/RConn1 -- Read_TimeInQueue/LConn1
  Start_TimeInSystem/RConn1 -- Start_TimeInQueue/LConn1
  Read_TimeInSystem/RConn1 -- Departures/RConn1
  Start_TimeInQueue/RConn1 -- FIFOQueue/LConn1
  SingleServer_WaitForRepair/LConn1 -- SingleServer_WaitForFailure/RConn1
  EventBasedEntityGen/RConn1 -- Path Combiner/LConn1
  Path Combiner/LConn2 -- SingleServer_WaitForRepair/RConn1
  Read_TimeInQueue/RConn1 -- N-Server/LConn1
  Arrivals/RConn1 -- Start_TimeInSystem/LConn1
  N-Server/RConn1 -- Read_TimeInSystem/LConn1
  Path Combiner/RConn1 -- SingleServer_WaitForFailure/LConn1

== system SingleWorkstationModelLibrary/GG1Workstation_RandomCountUntilNonpreempSetup/ComputeTH ==
  CurrentTime : Inport
  nDepartures : Inport  Port=2
  Derivative : Derivative
  Divide1 : Product  Inputs=/*
  Event to Timed Signal1 : EventToTimedSignal
  TH_average : Outport
  TH_samples : Outport  Port=2
  wires:
  CurrentTime/1 -> Divide1/1
  Event to Timed Signal1/1 -> Derivative/1, Divide1/2
  Divide1/1 -> TH_average/1
  Derivative/1 -> TH_samples/1
  nDepartures/1 -> Event to Timed Signal1/1

== system SingleWorkstationModelLibrary/GG1Workstation_RandomCountUntilNonpreempSetup/ComputeUandA ==
  CurrentTime : Inport
  nInFailServer : Inport  Port=2
  nInProcServer : Inport  Port=3
  Add : Sum
  Divide : Product  Inputs=/*
  Divide1 : Product  Inputs=/*
  Event to Timed Signal : EventToTimedSignal
  Event to Timed Signal1 : EventToTimedSignal
  Gain : Gain  Gain=-1
  Integrator : Integrator
  Integrator1 : Integrator
  Product : Product
  Subtract : Sum  Inputs=+-
  Util_average : Outport
  Avail_average : Outport  Port=2
  wires:
  Event to Timed Signal/1 -> Integrator/1, Product/1  "This value is 0 or 1"
  nInFailServer/1 -> Event to Timed Signal/1
  nInProcServer/1 -> Event to Timed Signal1/1
  Integrator/1 -> Subtract/2  "netDowntime"
  CurrentTime/1 -> Subtract/1, Divide1/1
  Divide/1 -> Util_average/1
  Subtract/1 -> Divide/1, Divide1/2  "netUptime"
  Integrator1/1 -> Divide/2  "netBusytime"
  Gain/1 -> Product/2
  Product/1 -> Add/1  "If 1 in the FailServer, then this value should be negative the number in the ProcServer, such that their sum is 0."
  Add/1 -> Integrator1/1  "This value is an adjusted number in the ProcServer (zero if one in the FailServer)"
  Event to Timed Signal1/1 -> Add/2, Gain/1
  Divide1/1 -> Avail_average/1

== system SingleWorkstationModelLibrary/GG1Workstation_RandomCountUntilNonpreempSetup/ComputeWIP ==
  nArrivals : Inport
  nDepartures : Inport  Port=2
  CurrentTime : Inport  Port=3
  Divide : Product  Inputs=*/
  Event to Timed Signal : EventToTimedSignal
  Integrator : Integrator
  Subtract : Sum  Inputs=+-
  WIP_samples : Outport
  WIP_average : Outport  Port=2
  wires:
  Subtract/1 -> WIP_samples/1, Event to Timed Signal/1
  Event to Timed Signal/1 -> Integrator/1
  Divide/1 -> WIP_average/1
  Integrator/1 -> Divide/1
  nArrivals/1 -> Subtract/1
  nDepartures/1 -> Subtract/2
  CurrentTime/1 -> Divide/2
